simulink model "1"  (R2013b)
settings: Solver=ode3  StartTime=0.0  StopTime=10.0  RelTol=1e-3
settings Model: Creator=NASA  LastModifiedBy=NASA

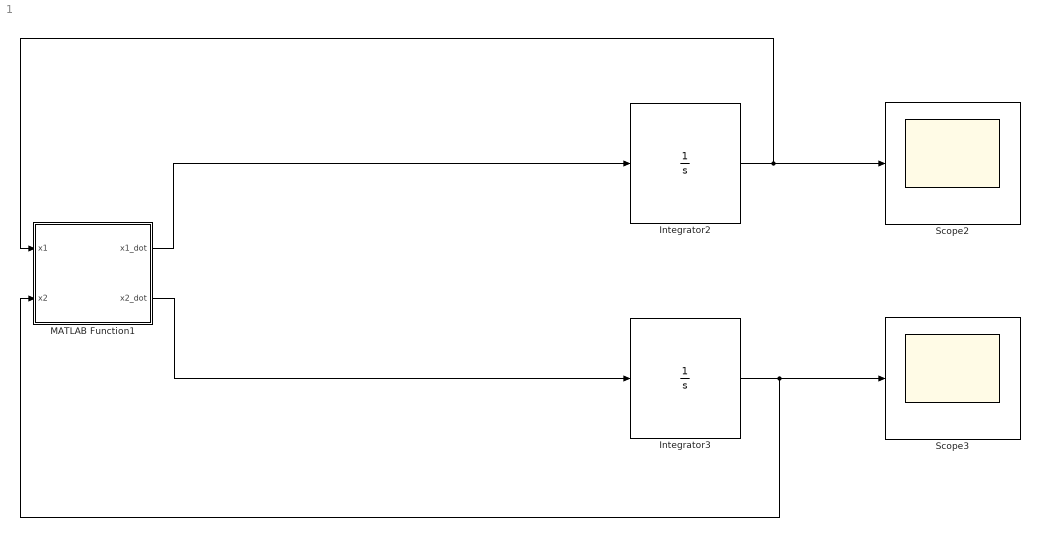
== system 1 ==
  Integrator2 : Integrator
  Integrator3 : Integrator
  MATLAB Function1 : MATLAB Function  TreatAsAtomicUnit=on
  Scope2 : Scope
      settings: SaveName=ScopeData2
  Scope3 : Scope
      settings: SaveName=ScopeData3
  wires:
  Integrator2/1 -> MATLAB Function1/1(x1), Scope2/1
  Integrator3/1 -> MATLAB Function1/2(x2), Scope3/1
  MATLAB Function1/2(x2_dot) -> Integrator3/1
  MATLAB Function1/1(x1_dot) -> Integrator2/1

== matlab function 1/MATLAB Function1 ==
  data: x1 input; x1_dot output; x2_dot output; x2 input
function [x1_dot, x2_dot]= fcn(x1,x2)
%#codegen

x1_dot = -x2 + 0.5*x1^3 + 0.5*x1*x2^2;
x2_dot = x1 + 0.5*x2*x1^2 + 0.5*x2^3;
